simulink model "MotionControlRobuFastObsDynWithPredAdams2"  (Simulink 7.1)
settings: Solver=ode23  StartTime=0.0  StopTime=50  MaxStep=0.002  MinStep=0.0001  RelTol=0.2  AbsTol=0.1
StartFcn:
  | parameters
StopFcn:
  | replay
values from neighbouring files (symbols this model uses):
  ADAMS_cwd = '/home/roland/Bureau/Simulateur/SimulateurAdamsFaizRobuFASTB2'    [Controls_Plant_1.m]
  ADAMS_exec = ''    [Controls_Plant_1.m]
  ADAMS_host = 'krid.isir.upmc.fr'    [Controls_Plant_1.m]
  ADAMS_init = ''    [Controls_Plant_1.m]
  ADAMS_inputs = 'AngleBraquageAV!AngleBraquageArriere!AccelMoteur!Stab_function'    [Controls_Plant_1.m]
  ADAMS_outputs = 'PosX!PosY!PosXAvant!PosYAvant!MesureVitesse!AngleAVG!AngleAVD!AngleARG!AngleARD!VitesseRoueARD!VitesseRoueARG!VitesseLacet!roulis'    [Controls_Plant_1.m]
  ADAMS_prefix = 'Controls_Plant_1'    [Controls_Plant_1.m]
  ADAMS_static = 'yes'    [Controls_Plant_1.m]
  ADAMS_sysdir = '/home/roland/Adams/'    [Controls_Plant_1.m]
  C = ParDyn(9)    [MvtDyn.m]    (also in ParPneu.m = 1.3; Replay.m = line([X_trac(6) X_trac(8)],[Y_trac(6) Y_trac(8)],'LineWidth')
  Corr180 = Angle    [corr180.m]
undefined symbols (not defined in the file or in its folder): braquage2train2Arr, braquage3train2, CalculHorizonPred, courbure, DetDyn, ecarts, Empattement, MdresCarres, ObsCFCRMITtrain2, ObsDynTrain2, point_plus_proche, TrouvePos, Voie
libraries: simulink x8
(part 2 of 2)

== system MotionControlRobuFastObsDynWithPredAdams2/ExtractionEtat/Retard2/Corr1 ==
  In1 : Inport
  MATLAB Fcn : MATLABFcn  MATLABFcn=Corr180(u(1))  OutputDimensions=1  SampleTime=0.05
  Out1 : Outport
  wires:
  In1/1 -> MATLAB Fcn/1
  MATLAB Fcn/1 -> Out1/1

== system MotionControlRobuFastObsDynWithPredAdams2/ExtractionEtat/Retard2/CorrPente ==
  In1 : Inport
  Divide3 : Product  Inputs=*/  OutDataType=sfix(16)  OutScaling=2^-10
  Trigonometric Function2 : Trigonometry  Operator=cos
  Out1 : Outport
  wires:
  In1/1 -> Divide3/1
  [Roulis] -> Trigonometric Function2/1
  Trigonometric Function2/1 -> Divide3/2
  Divide3/1 -> Out1/1

== system MotionControlRobuFastObsDynWithPredAdams2/RobuFAST1/adams_sub/ADAMS Plant ==
  ADAMS inputs : Inport
  S-Function : S-Function  FunctionName=adams_plant  Parameters=exevie,exesol,stat,outfil,nampre,o_rate,nam_in,namout,dft,modsim,modani,dt_out,inicmd,exetyp,comtyp,ada_host, workdir,interorder  EnableBusSupport=off
  ADAMS outputs : Outport  InitialOutput=0
  wires:
  ADAMS inputs/1 -> S-Function/1
  S-Function/1 -> ADAMS outputs/1
